simulink library "environment"  (R2021b)
settings: Solver=VariableStepAuto  StartTime=0.0  StopTime=10.0  RelTol=1e-3
undefined symbols (not defined in the file or in its folder): a, A_i, alfaG, Cd, g, H, h, h0, hmax, J, k, mu, N_i, n_sun, N_sur, om_Earth, P, r_i, rho0, rho_d, rho_s, Rt
libraries: my_math_ops x5, matrix_library x4, simulink x3, ctransform x1
settings Model: Creator=Davide  LastModifiedBy=Davide

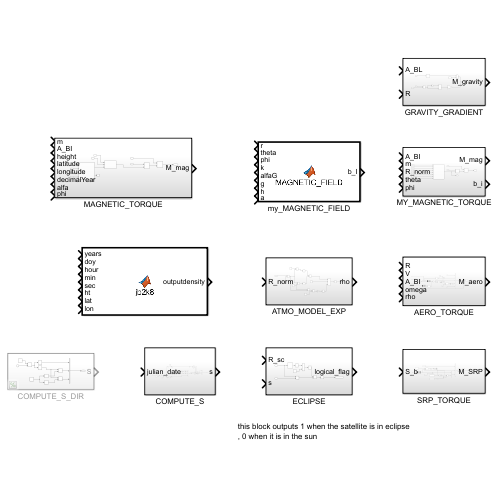
[thumbnail: Simulink's stored preview of the top-level diagram]
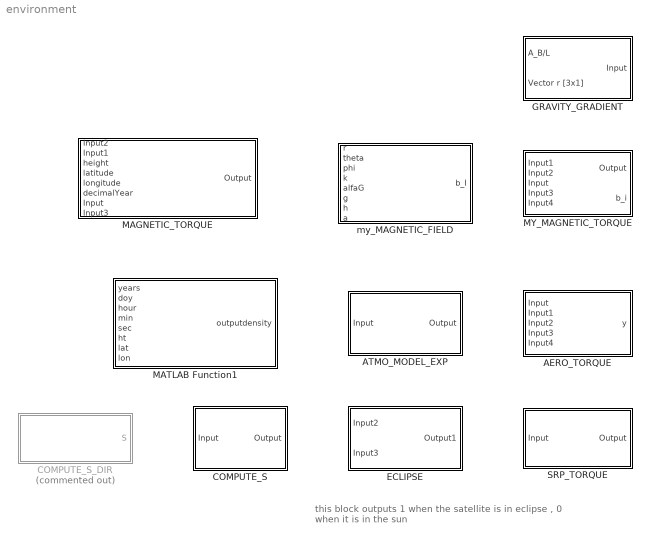
== system environment ==
  note: this block outputs 1 when the satellite is in eclipse
      | , 0 when it is in the sun
  AERO_TORQUE : Subsystem
  ATMO_MODEL_EXP : Subsystem
  COMPUTE_S : Subsystem
  COMPUTE_S_DIR : Subsystem  Commented=on
  ECLIPSE : Subsystem
  GRAVITY_GRADIENT : Subsystem
  MAGNETIC_TORQUE : Subsystem
  MATLAB Function1 : MATLAB Function  TreatAsAtomicUnit=on
  MY_MAGNETIC_TORQUE : Subsystem
  SRP_TORQUE : Subsystem
  my_MAGNETIC_FIELD : MATLAB Function  TreatAsAtomicUnit=on

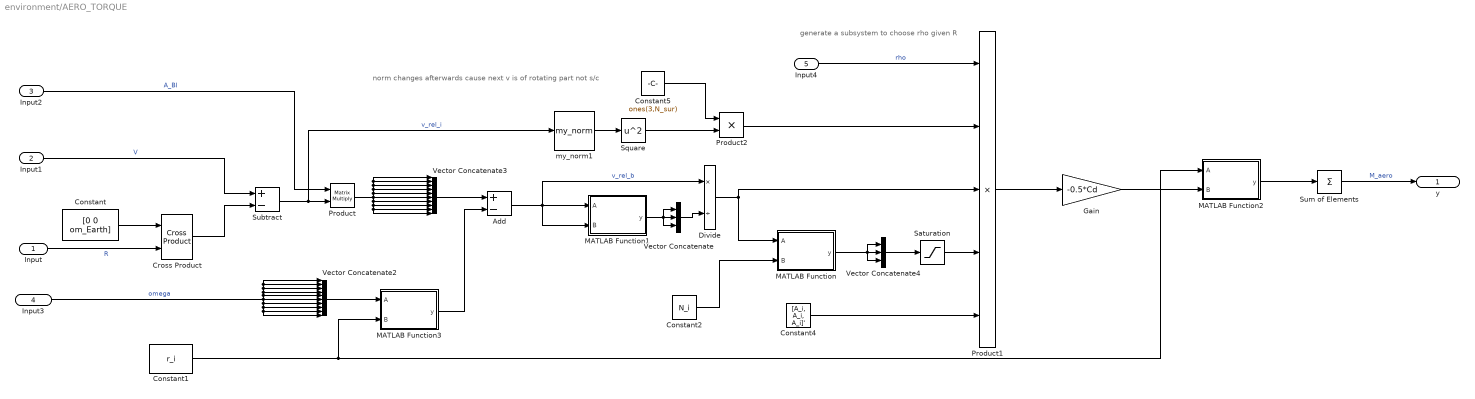
== system environment/AERO_TORQUE ==
  note: norm changes afterwards cause next v is of rotating part not s/c
  note: generate a subsystem to choose rho given R
  Input : Inport
  Input1 : Inport  Port=2
  Input2 : Inport  Port=3
  Input3 : Inport  Port=4
  Input4 : Inport  Port=5
  Add : Sum  Inputs=+-
  Constant : Constant  Value=[0 0 om_Earth]
  Constant1 : Constant  Value=r_i
  Constant2 : Constant  Value=N_i
  Constant4 : Constant  Value=[A_i, A_i, A_i]'
  Constant5 : Constant  Value=ones(3,N_sur)
  Cross Product : matrix_library/Cross Product
      settings: SourceProductBaseCode=SL
  Divide : Product  Inputs=*/
  Gain : Gain  Gain=-0.5*Cd
  MATLAB Function : MATLAB Function  TreatAsAtomicUnit=on
  MATLAB Function1 : MATLAB Function  TreatAsAtomicUnit=on
  MATLAB Function2 : MATLAB Function  TreatAsAtomicUnit=on
  MATLAB Function3 : MATLAB Function  TreatAsAtomicUnit=on
  Product : Product  Multiplication=Matrix(*)
  Product1 : Product  Inputs=5
  Product2 : Product
  Saturation : Saturate  UpperLimit=inf  LowerLimit=0
  Square : Math  Operator=square  SaturateOnIntegerOverflow=on
  Subtract : Sum  Inputs=+-
  Sum of Elements : Sum  Inputs=+  CollapseMode=Specified dimension  CollapseDim=2
  Vector Concatenate : Concatenate  NumInputs=3  Mode=Multidimensional array
  Vector Concatenate2 : Concatenate  NumInputs=N_sur  Mode=Multidimensional array  ConcatenateDimension=2
  Vector Concatenate3 : Concatenate  NumInputs=N_sur  Mode=Multidimensional array  ConcatenateDimension=2
  Vector Concatenate4 : Concatenate  NumInputs=3  Mode=Multidimensional array
  my_norm1 : my_math_ops/my_norm  SystemSampleTime=-1  VariantActivationTime=update diagram  Latency=0  AutoFrameSizeCalculation=off
      settings: SourceProductName=My Mathematics Operations
  y : Outport
  wires:
  Vector Concatenate4/1 -> Saturation/1
  MATLAB Function/1(y) -> Vector Concatenate4/2, Vector Concatenate4/1, Vector Concatenate4/3
  Sum of Elements/1 -> y/1  "M_aero"
  Vector Concatenate/1 -> Divide/2
  MATLAB Function1/1(y) -> Vector Concatenate/2, Vector Concatenate/3, Vector Concatenate/1
  Vector Concatenate3/1 -> Add/1
  Product/1 -> Vector Concatenate3/6, Vector Concatenate3/7, Vector Concatenate3/8, Vector Concatenate3/9, Vector Concatenate3/10, Vector Concatenate3/1, Vector Concatenate3/2, Vector Concatenate3/3, Vector Concatenate3/4, Vector Concatenate3/5
  Vector Concatenate2/1 -> MATLAB Function3/1(A)
  Input3/1 -> Vector Concatenate2/6, Vector Concatenate2/7, Vector Concatenate2/8, Vector Concatenate2/9, Vector Concatenate2/10, Vector Concatenate2/1, Vector Concatenate2/2, Vector Concatenate2/3, Vector Concatenate2/4, Vector Concatenate2/5  "omega"
  Product2/1 -> Product1/2
  Constant5/1 -> Product2/1
  MATLAB Function2/1(y) -> Sum of Elements/1
  Cross Product/1 -> Subtract/2
  Input2/1 -> Product/1  "A_BI"
  Subtract/1 -> my_norm1/1, Product/2  "v_rel_i"
  Gain/1 -> MATLAB Function2/2(B)
  Input1/1 -> Subtract/1  "V"
  Product1/1 -> Gain/1
  Input/1 -> Cross Product/2  "R"
  MATLAB Function3/1(y) -> Add/2
  Square/1 -> Product2/2
  Constant/1 -> Cross Product/1
  my_norm1/1 -> Square/1
  Add/1 -> MATLAB Function1/1(A), MATLAB Function1/2(B), Divide/1  "v_rel_b"
  Input4/1 -> Product1/1  "rho"
  Divide/1 -> Product1/3, MATLAB Function/1(A)
  Constant2/1 -> MATLAB Function/2(B)
  Constant4/1 -> Product1/5
  Saturation/1 -> Product1/4
  Constant1/1 -> MATLAB Function3/2(B), MATLAB Function2/1(A)

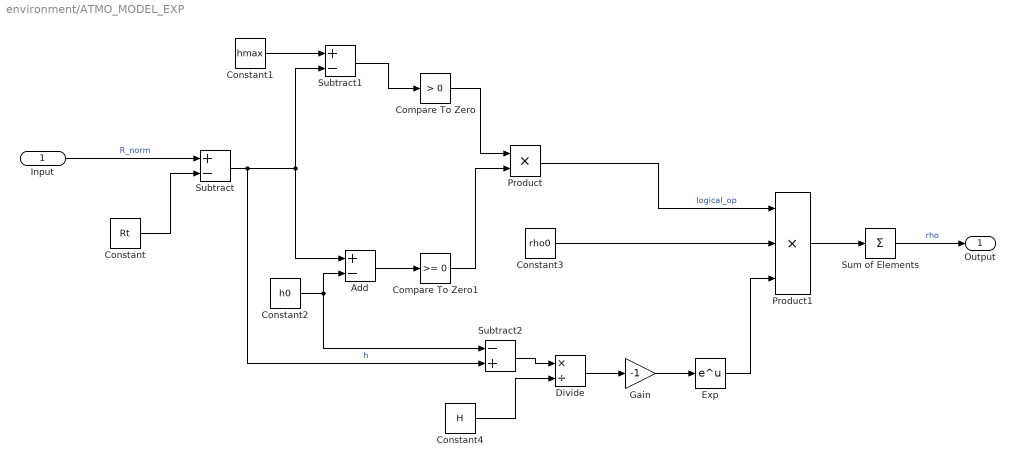
== system environment/ATMO_MODEL_EXP ==
  Input : Inport
  Add : Sum  Inputs=+-
  Compare To Zero : simulink/Logic and Bit Operations/Compare To Zero  relop=>  OutDataTypeStr=boolean
  Compare To Zero1 : simulink/Logic and Bit Operations/Compare To Zero  relop=>=  OutDataTypeStr=boolean
  Constant : Constant  Value=Rt
  Constant1 : Constant  Value=hmax
  Constant2 : Constant  Value=h0
  Constant3 : Constant  Value=rho0
  Constant4 : Constant  Value=H
  Divide : Product  Inputs=*/
  Exp : Math  SaturateOnIntegerOverflow=on
  Gain : Gain  Gain=-1
  Product : Product
  Product1 : Product  Inputs=3
  Subtract : Sum  Inputs=+-
  Subtract1 : Sum  Inputs=+-
  Subtract2 : Sum  Inputs=-+
  Sum of Elements : Sum  Inputs=+
  Output : Outport
  wires:
  Constant/1 -> Subtract/2
  Input/1 -> Subtract/1  "R_norm"
  Subtract/1 -> Subtract2/2, Add/1, Subtract1/2  "h"
  Constant1/1 -> Subtract1/1
  Subtract1/1 -> Compare To Zero/1
  Constant2/1 -> Subtract2/1, Add/2
  Add/1 -> Compare To Zero1/1
  Compare To Zero/1 -> Product/1
  Compare To Zero1/1 -> Product/2
  Product/1 -> Product1/1  "logical_op"
  Constant3/1 -> Product1/2
  Constant4/1 -> Divide/2
  Subtract2/1 -> Divide/1
  Divide/1 -> Gain/1
  Gain/1 -> Exp/1
  Exp/1 -> Product1/3
  Product1/1 -> Sum of Elements/1
  Sum of Elements/1 -> Output/1  "rho"

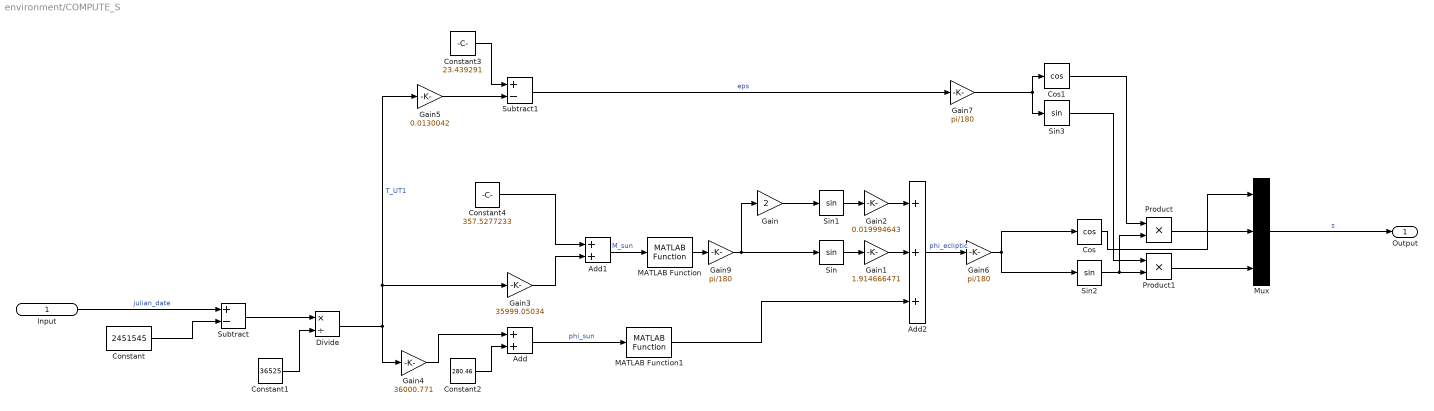
== system environment/COMPUTE_S ==
  Input : Inport
  Add : Sum
  Add1 : Sum
  Add2 : Sum  Inputs=+++
  Constant : Constant  Value=2451545
  Constant1 : Constant  Value=36525
  Constant2 : Constant  Value=280.46
  Constant3 : Constant  Value=23.439291
  Constant4 : Constant  Value=357.5277233
  Cos : Trigonometry  Operator=cos
  Cos1 : Trigonometry  Operator=cos
  Divide : Product  Inputs=*/
  Gain : Gain  Gain=2
  Gain1 : Gain  Gain=1.914666471
  Gain2 : Gain  Gain=0.019994643
  Gain3 : Gain  Gain=35999.05034
  Gain4 : Gain  Gain=36000.771
  Gain5 : Gain  Gain=0.0130042
  Gain6 : Gain  Gain=pi/180
  Gain7 : Gain  Gain=pi/180
  Gain9 : Gain  Gain=pi/180
  MATLAB Function : my_math_ops/MATLAB Function  SystemSampleTime=-1  VariantActivationTime=update diagram  Latency=0  AutoFrameSizeCalculation=off
  MATLAB Function1 : my_math_ops/MATLAB Function  SystemSampleTime=-1  VariantActivationTime=update diagram  Latency=0  AutoFrameSizeCalculation=off
  Mux : Mux  Inputs=3
  Product : Product
  Product1 : Product
  Sin{,1..3} (4 alike) : Trigonometry
  Subtract : Sum  Inputs=+-
  Subtract1 : Sum  Inputs=+-
  Output : Outport
  wires:
  Constant3/1 -> Subtract1/1
  Gain5/1 -> Subtract1/2
  Cos1/1 -> Product/1
  Mux/1 -> Output/1  "s"
  Sin3/1 -> Product1/1
  Product1/1 -> Mux/3
  Sin2/1 -> Product1/2, Product/2
  Constant/1 -> Subtract/2
  Divide/1 -> Gain4/1, Gain5/1, Gain3/1  "T_UT1"
  Add1/1 -> MATLAB Function/1  "M_sun"
  Gain1/1 -> Add2/2
  Gain2/1 -> Add2/1
  Add2/1 -> Gain6/1  "phi_ecliptic"
  Constant4/1 -> Add1/1
  Gain6/1 -> Cos/1, Sin2/1
  Gain7/1 -> Cos1/1, Sin3/1
  Constant2/1 -> Add/2
  Subtract/1 -> Divide/1
  Add/1 -> MATLAB Function1/1  "phi_sun"
  Input/1 -> Subtract/1  "julian_date"
  Constant1/1 -> Divide/2
  Sin1/1 -> Gain2/1
  Gain3/1 -> Add1/2
  Product/1 -> Mux/2
  Gain4/1 -> Add/1
  Sin/1 -> Gain1/1
  Cos/1 -> Mux/1
  Subtract1/1 -> Gain7/1  "eps"
  Gain/1 -> Sin1/1
  Gain9/1 -> Sin/1, Gain/1
  MATLAB Function/1 -> Gain9/1
  MATLAB Function1/1 -> Add2/3

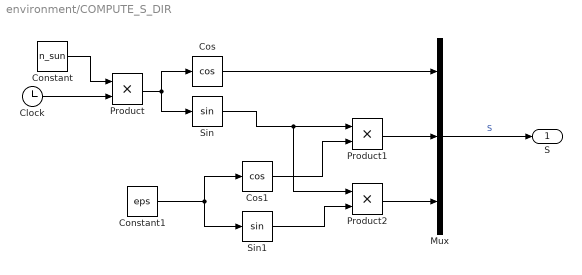
== system environment/COMPUTE_S_DIR ==
  Clock : Clock
  Constant : Constant  Value=n_sun
  Constant1 : Constant  Value=eps
  Cos : Trigonometry  Operator=cos
  Cos1 : Trigonometry  Operator=cos
  Mux : Mux  Inputs=3
  Product : Product
  Product1 : Product
  Product2 : Product
  Sin : Trigonometry
  Sin1 : Trigonometry
  S : Outport
  wires:
  Product2/1 -> Mux/3
  Sin/1 -> Product2/1, Product1/1
  Product/1 -> Sin/1, Cos/1
  Constant1/1 -> Sin1/1, Cos1/1
  Constant/1 -> Product/1
  Cos1/1 -> Product1/2
  Sin1/1 -> Product2/2
  Clock/1 -> Product/2
  Product1/1 -> Mux/2
  Cos/1 -> Mux/1
  Mux/1 -> S/1  "S"

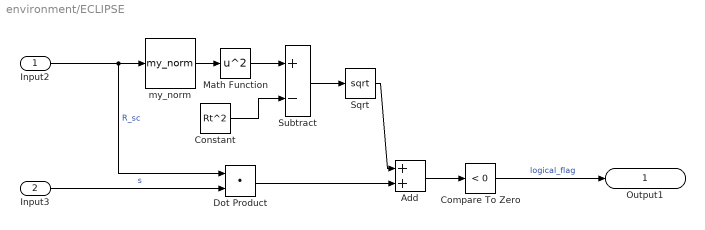
== system environment/ECLIPSE ==
  Input2 : Inport
  Input3 : Inport  Port=2
  Add : Sum
  Compare To Zero : simulink/Logic and Bit Operations/Compare To Zero  relop=<  OutDataTypeStr=boolean
  Constant : Constant  Value=Rt^2
  Dot Product : DotProduct  InputSameDT=on  OutDataTypeStr=Inherit: Inherit via internal rule
  Math Function : Math  Operator=square  SaturateOnIntegerOverflow=on
  Sqrt : Sqrt  SaturateOnIntegerOverflow=on
  Subtract : Sum  Inputs=+-
  my_norm : my_math_ops/my_norm  SystemSampleTime=-1  VariantActivationTime=update diagram  Latency=0  AutoFrameSizeCalculation=off
      settings: SourceProductName=My Mathematics Operations
  Output1 : Outport
  wires:
  Subtract/1 -> Sqrt/1
  Input3/1 -> Dot Product/2  "s"
  Sqrt/1 -> Add/1
  Dot Product/1 -> Add/2
  Add/1 -> Compare To Zero/1
  Constant/1 -> Subtract/2
  my_norm/1 -> Math Function/1
  Input2/1 -> Dot Product/1, my_norm/1  "R_sc"
  Compare To Zero/1 -> Output1/1  "logical_flag"
  Math Function/1 -> Subtract/1

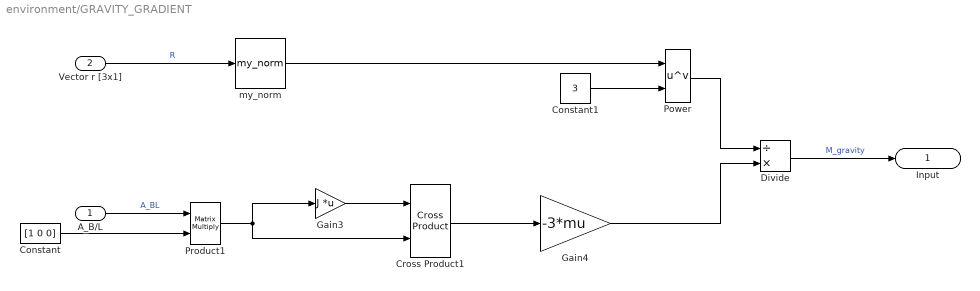
== system environment/GRAVITY_GRADIENT ==
  A_B/L : Inport
  Vector r [3x1] : Inport  Port=2
  Constant : Constant  Value=[1 0 0]
  Constant1 : Constant  Value=3
  Cross Product1 : matrix_library/Cross Product
      settings: SourceProductBaseCode=SL
  Divide : Product  Inputs=/*
  Gain3 : Gain  Gain=J  Multiplication=Matrix(K*u)
  Gain4 : Gain  Gain=-3*mu
  Power : Math  Operator=pow  SaturateOnIntegerOverflow=on
  Product1 : Product  Multiplication=Matrix(*)
  my_norm : my_math_ops/my_norm  SystemSampleTime=-1  VariantActivationTime=update diagram  Latency=0  AutoFrameSizeCalculation=off
      settings: SourceProductName=My Mathematics Operations
  Input : Outport
  wires:
  Vector r [3x1]/1 -> my_norm/1  "R"
  A_B/L/1 -> Product1/1  "A_BL"
  Cross Product1/1 -> Gain4/1
  Power/1 -> Divide/1
  Gain4/1 -> Divide/2
  Product1/1 -> Cross Product1/2, Gain3/1
  Constant/1 -> Product1/2
  Constant1/1 -> Power/2
  Gain3/1 -> Cross Product1/1
  Divide/1 -> Input/1  "M_gravity"
  my_norm/1 -> Power/1

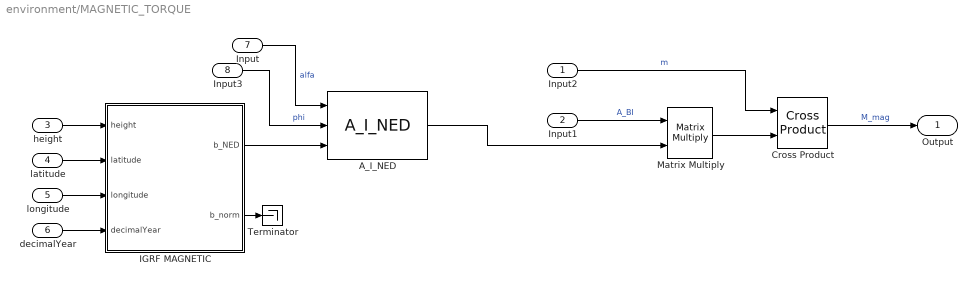
== system environment/MAGNETIC_TORQUE ==
  Input2 : Inport
  Input1 : Inport  Port=2
  height : Inport  Port=3
  latitude : Inport  Port=4
  longitude : Inport  Port=5
  decimalYear : Inport  Port=6
  Input : Inport  Port=7
  Input3 : Inport  Port=8
  A_I_NED : ctransform/A_I_NED  SystemSampleTime=-1  VariantActivationTime=update diagram  Latency=0  AutoFrameSizeCalculation=off
      settings: SourceProductName=Frame Transformations
  Cross Product : matrix_library/Cross Product
      settings: SourceProductBaseCode=SL
  IGRF MAGNETIC : MATLAB Function  TreatAsAtomicUnit=on
  Matrix Multiply : Product  Multiplication=Matrix(*)
  Terminator : Terminator
  Output : Outport
  wires:
  Input1/1 -> Matrix Multiply/1  "A_BI"
  Cross Product/1 -> Output/1  "M_mag"
  Matrix Multiply/1 -> Cross Product/2
  latitude/1 -> IGRF MAGNETIC/2(latitude)
  A_I_NED/1 -> Matrix Multiply/2
  Input2/1 -> Cross Product/1  "m"
  longitude/1 -> IGRF MAGNETIC/3(longitude)
  height/1 -> IGRF MAGNETIC/1(height)
  IGRF MAGNETIC/2(b_norm) -> Terminator/1
  IGRF MAGNETIC/1(b_NED) -> A_I_NED/3
  decimalYear/1 -> IGRF MAGNETIC/4(decimalYear)
  Input/1 -> A_I_NED/1  "alfa"
  Input3/1 -> A_I_NED/2  "phi"

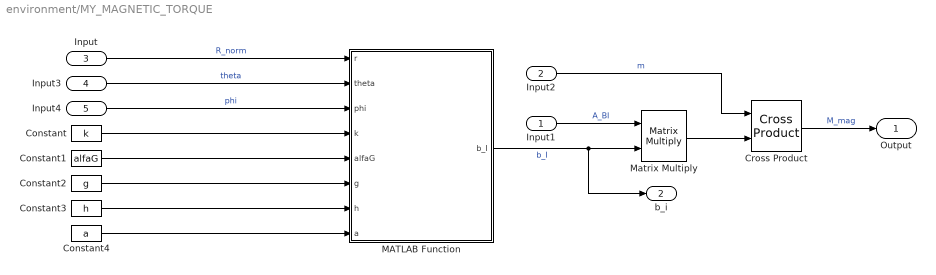
== system environment/MY_MAGNETIC_TORQUE ==
  Input1 : Inport
  Input2 : Inport  Port=2
  Input : Inport  Port=3
  Input3 : Inport  Port=4
  Input4 : Inport  Port=5
  Constant : Constant  Value=k
  Constant1 : Constant  Value=alfaG
  Constant2 : Constant  Value=g
  Constant3 : Constant  Value=h
  Constant4 : Constant  Value=a
  Cross Product : matrix_library/Cross Product
      settings: SourceProductBaseCode=SL
  MATLAB Function : MATLAB Function  TreatAsAtomicUnit=on
  Matrix Multiply : Product  Multiplication=Matrix(*)
  Output : Outport
  b_i : Outport  Port=2
  wires:
  Input2/1 -> Cross Product/1  "m"
  Matrix Multiply/1 -> Cross Product/2
  MATLAB Function/1(b_I) -> b_i/1, Matrix Multiply/2  "b_I"
  Input1/1 -> Matrix Multiply/1  "A_BI"
  Cross Product/1 -> Output/1  "M_mag"
  Constant/1 -> MATLAB Function/4(k)
  Constant1/1 -> MATLAB Function/5(alfaG)
  Constant2/1 -> MATLAB Function/6(g)
  Constant4/1 -> MATLAB Function/8(a)
  Constant3/1 -> MATLAB Function/7(h)
  Input/1 -> MATLAB Function/1(r)  "R_norm"
  Input3/1 -> MATLAB Function/2(theta)  "theta"
  Input4/1 -> MATLAB Function/3(phi)  "phi"

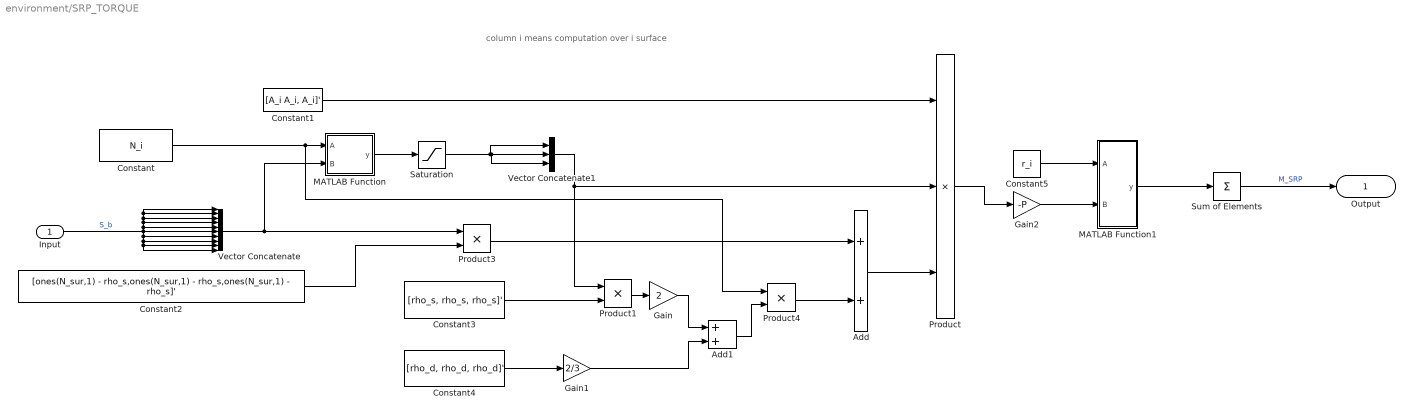
== system environment/SRP_TORQUE ==
  note: column i means computation over i surface
  Input : Inport
  Add : Sum
  Add1 : Sum
  Constant : Constant  Value=N_i
  Constant1 : Constant  Value=[A_i A_i, A_i]'
  Constant2 : Constant  Value=[ones(N_sur,1) - rho_s,ones(N_sur,1) - rho_s,ones(N_sur,1) - rho_s]'  VectorParams1D=off
  Constant3 : Constant  Value=[rho_s, rho_s, rho_s]'
  Constant4 : Constant  Value=[rho_d, rho_d, rho_d]'
  Constant5 : Constant  Value=r_i
  Gain : Gain  Gain=2
  Gain1 : Gain  Gain=2/3
  Gain2 : Gain  Gain=-P
  MATLAB Function : MATLAB Function  TreatAsAtomicUnit=on
  MATLAB Function1 : MATLAB Function  TreatAsAtomicUnit=on
  Product : Product  Inputs=3
  Product1 : Product
  Product3 : Product
  Product4 : Product
  Saturation : Saturate  UpperLimit=inf  LowerLimit=0
  Sum of Elements : Sum  Inputs=+  CollapseMode=Specified dimension  CollapseDim=2
  Vector Concatenate : Concatenate  NumInputs=N_sur  Mode=Multidimensional array  ConcatenateDimension=2
  Vector Concatenate1 : Concatenate  NumInputs=3  Mode=Multidimensional array
  Output : Outport
  wires:
  Input/1 -> Vector Concatenate/1, Vector Concatenate/2, Vector Concatenate/3, Vector Concatenate/4, Vector Concatenate/5, Vector Concatenate/6, Vector Concatenate/7, Vector Concatenate/9, Vector Concatenate/10, Vector Concatenate/8  "S_b"
  Add1/1 -> Product4/2
  MATLAB Function1/1(y) -> Sum of Elements/1
  Vector Concatenate1/1 -> Product1/1, Product/2
  Constant/1 -> Product4/1, MATLAB Function/1(A)
  Saturation/1 -> Vector Concatenate1/1, Vector Concatenate1/3, Vector Concatenate1/2
  Sum of Elements/1 -> Output/1  "M_SRP"
  Constant1/1 -> Product/1
  Product4/1 -> Add/2
  Gain/1 -> Add1/1
  Gain1/1 -> Add1/2
  Vector Concatenate/1 -> MATLAB Function/2(B), Product3/1
  MATLAB Function/1(y) -> Saturation/1
  Product/1 -> Gain2/1
  Constant2/1 -> Product3/2
  Product1/1 -> Gain/1
  Constant3/1 -> Product1/2
  Product3/1 -> Add/1
  Constant4/1 -> Gain1/1
  Add/1 -> Product/3
  Constant5/1 -> MATLAB Function1/1(A)
  Gain2/1 -> MATLAB Function1/2(B)

== matlab function environment/MATLAB Function1 ==
  data: years input; doy input; hour input; min input; sec input; ht input; lat input; lon input; outputdensity output
function outputdensity  = jb2k8(years,doy,hour,min,sec,ht,lat,lon)

% JB2008 Calling Script.
% jb2k8 is used to call the JB2008 model in MATLAB. It can also be embedded
% in a SIMULINK block if desired.
%
% Replace any outputs with a ~ to skip them.
% [~,~,~,~,~,~,~,~,~,~,~,~,outputdensity,~,~,~,~,~,~,~,~,~,~] = jb2k8(years,doy,hour,min,sec,ht,lat,lon)
%
%
%



%% Check for latest version and all required files.
% The sum of the "exist" results should add to 8.

FileSum = exist('SOLFSMY.TXT') + exist('SOLRESAP.TXT') + ...
 exist('DSTFILE.TXT') +  exist('DTCFILE.TXT');

if  verLessThan('matlab', '8.4') == 1 & FileSum == 8
    disp(['MATLAB 2014b or later is required to automatically update files.'])
    disp(['Files may be out of date!'])
end


%% Update required text files if necessary

UpdateFile('SOLFSMY.TXT');
UpdateFile('DTCFILE.TXT');
UpdateFile('DSTFILE.TXT');
UpdateFile('SOLRESAP.TXT');

%% Check the the input date is not later than the latest date of the input files.

% doytoday = datenum(date) - datenum(year(date),1,1) + 1;
% 
% if years >= year(date) & doy >= doytoday
%     disp(['Choose another date.'])
% return
% end

%% Call the JB2008 function

formatSpec = 'JB2008.exe%5d%5d%5d%5d%7.3f%9.2f%8.2f%8.2f';
inputdata = sprintf(formatSpec,years,doy,hour,min,sec,ht,lat,lon);

[status,cmdout] = system(inputdata);

G = textscan(cmdout,'%f %f %f %f %f %f %f %f %f %f %f %f %f %f %f %f %f %f %f %f %f %f %f');


%% Outputs
outputs1 = G{1,1};
% outputs2 = G{1,2};

% % Time
%     outputyear = outputs1(1);
%     outputdoy = outputs1(2);
%     outputhr = outputs1(3);
%     outputmin = outputs1(4);
%     outputsec = outputs1(5);
% % Location
%     outputht = outputs1(6);
%     outputlat = outputs1(7);
%     outputlon = outputs1(8);
% % Misc
%     outputsun1 = outputs1(9);
%     outputsun2 = outputs2(9);
%     outputtemp1 = outputs1(10);
%     outputtemp2 = outputs2(10);

% Density
    outputdensity  = outputs1(11);

% Indices
%     outputD1950 = outputs1(12);
%     outputF10 = outputs1(13);
%     outputF10B = outputs1(14);
%     outputS10 = outputs1(15);
%     outputS10B = outputs1(16);
%     outputXM10 = outputs1(17);
%     outputXM10B = outputs1(18);
%     outputY10 = outputs1(19);
%     outputY10B = outputs1(20);
%     outputDSTDTC = outputs1(21);

== matlab function environment/MAGNETIC_TORQUE/IGRF MAGNETIC ==
  data: height input; b_NED output; latitude input; longitude input; decimalYear input; b_norm output
function [b_NED,b_norm] = fun(height,latitude,longitude,decimalYear)
%returns magnetic field in nT and NED reference frame
[b_NED,~,~,b_norm,~,~,~,~,~,~] = igrfmagm(height,latitude,longitude,decimalYear);

== matlab function environment/SRP_TORQUE/MATLAB Function ==
  data: A input; y output; B input
function y = fcn(A,B)
y = dot(A,B);

== matlab function environment/MY_MAGNETIC_TORQUE/MATLAB Function ==
  data: r input; b_I output; theta input; phi input; k input; alfaG input; g input; h input; a input
function b_I = MAGNETIC_FIELD(r,theta,phi,k,alfaG,g,h,a)
%calculate in ECI coordinates the Earth magnetic field b via a spherical
%harmonic model (quasi-Schmidt normalized formulas)
%
% PROTOTYPE:
%   b_I = MAGNETIC_FIELD(r,theta,phi,k,alfaG,g,h,R)
%
% INPUT:
%    r[-]            radius at which b is computed [Km]
%    theta[-]        latitude at which b is computed [rad]
%    phi[-]          longitude at which Pnm is calculated [rad]
%    k[-]            order of the model
%    alfaG[-]        initial longitude of observer meridian [rad]
%	 g[13x14] 	     first gaussian coefficent (n->rows ,m->columns) [T]
%	 h[13x14] 	     second gaussian coefficent (n->rows ,m->columns) [T]
%    a[-]            reference radius of the Earth [from paper 6371.2 Km]
%
% OUTPUT:
%	 b_I[3x1] 	     Earth magnetic field in ECI coordinates
%
% CONTRIBUTORS:
%   Davide Zamblera - Politecnico di Milano - Space eng.
%
% VERSIONS
% 2021-11-06: First version
%
b_r = 0;
b_th = 0;
b_phi = 0;
theta = pi/2 - theta;
[P,dP] = coeffP(k,theta);
P = P(2:end,:);
dP = dP(2:end,:);
for n = 1:k
    s1 = 0;
    s2 = 0;
    s3 = 0;
    for m = 0:n
        s1 = s1 + (g(n,m+1) * cos(m*phi) + h(n,m+1) * sin(m*phi)) * P(n,m+1);
        s2 = s2 + (g(n,m+1) * cos(m*phi) + h(n,m+1) * sin(m*phi)) * dP(n,m+1);
        s3 = s3 + m*(-g(n,m+1) * sin(m*phi) + h(n,m+1) * cos(m*phi)) * P(n,m+1);
    end
    b_r = b_r + (a/r)^(n+2) * (n+1) * s1;
    b_th = b_th + (a/r)^(n+2) * s2;
    b_phi = b_phi + (a/r)^(n+2) * s3;
end
b_th = - b_th;
b_phi = -1/sin(theta) * b_phi;

delta = pi/2 - theta;
alfa = phi + alfaG;

b1 = (b_r * cos(delta) + b_th * sin(delta))*cos(alfa) - b_phi * sin(alfa);
b2 = (b_r*cos(delta)+b_th*sin(delta))*sin(alfa)+b_phi*cos(alfa);
b3 = (b_r*sin(delta) - b_th*cos(delta));
b_I = [b1,b2,b3]';
end

== matlab function environment/SRP_TORQUE/MATLAB Function1 ==
  data: A input; y output; B input
function y = fcn(A,B)
y = cross(A,B);

== matlab function environment/AERO_TORQUE/MATLAB Function ==
  data: A input; y output; B input
function y = fcn(A,B)

y = dot(A,B);

== matlab function environment/AERO_TORQUE/MATLAB Function1 ==
  data: A input; y output; B input
function y = fcn(A,B)

y = dot(A,B);

== matlab function environment/AERO_TORQUE/MATLAB Function2 ==
  data: A input; y output; B input
function y = fcn(A,B)

y = cross(A,B);

== matlab function environment/AERO_TORQUE/MATLAB Function3 ==
  data: A input; y output; B input
function y = fcn(A,B)

y = cross(A,B);

== matlab function environment/my_MAGNETIC_FIELD ==
  data: r input; b_I output; theta input; phi input; k input; alfaG input; g input; h input; a input
function b_I = MAGNETIC_FIELD(r,theta,phi,k,alfaG,g,h,a)
%calculate in ECI coordinates the Earth magnetic field b via a spherical
%harmonic model (quasi-Schmidt normalized formulas)
%
% PROTOTYPE:
%   b_I = MAGNETIC_FIELD(r,theta,phi,k,alfaG,g,h,R)
%
% INPUT:
%    r[-]            radius at which b is computed [Km]
%    theta[-]        latitude at which b is computed [rad]
%    phi[-]          longitude at which Pnm is calculated [rad]
%    k[-]            order of the model
%    alfaG[-]        initial longitude of observer meridian [rad]
%	 g[13x14] 	     first gaussian coefficent (n->rows ,m->columns) [T]
%	 h[13x14] 	     second gaussian coefficent (n->rows ,m->columns) [T]
%    a[-]            reference radius of the Earth [from paper 6371.2 Km]
%
% OUTPUT:
%	 b_I[3x1] 	     Earth magnetic field in ECI coordinates
%
% CONTRIBUTORS:
%   Davide Zamblera - Politecnico di Milano - Space eng.
%
% VERSIONS
% 2021-11-06: First version
%
b_r = 0;
b_th = 0;
b_phi = 0;
theta = pi/2 - theta;
[P,dP] = coeffP(k,theta);
P = P(2:end,:);
dP = dP(2:end,:);
for n = 1:k
    s1 = 0;
    s2 = 0;
    s3 = 0;
    for m = 0:n
        s1 = s1 + (g(n,m+1) * cos(m*phi) + h(n,m+1) * sin(m*phi)) * P(n,m+1);
        s2 = s2 + (g(n,m+1) * cos(m*phi) + h(n,m+1) * sin(m*phi)) * dP(n,m+1);
        s3 = s3 + m*(-g(n,m+1) * sin(m*phi) + h(n,m+1) * cos(m*phi)) * P(n,m+1);
    end
    b_r = b_r + (a/r)^(n+2) * (n+1) * s1;
    b_th = b_th + (a/r)^(n+2) * s2;
    b_phi = b_phi + (a/r)^(n+2) * s3;
end
b_th = - b_th;
b_phi = -1/sin(theta) * b_phi;

delta = pi/2 - theta;
alfa = phi + alfaG;

b1 = (b_r * cos(delta) + b_th * sin(delta))*cos(alfa) - b_phi * sin(alfa);
b2 = (b_r*cos(delta)+b_th*sin(delta))*sin(alfa)+b_phi*cos(alfa);
b3 = (b_r*sin(delta) - b_th*cos(delta));
b_I = [b1,b2,b3]';
end
